simulink model "wind_turbine_modified"  (R2023a)
settings: Solver=VariableStepAuto  StartTime=0.0  StopTime=10.0  RelTol=1e-3
undefined symbols (not defined in the file): F, find_system, Fnom, gcbh, H, ILd_init, ILq_init, Imax_grid_conv, Init, j, Ki_dc_reg, Ki_grid_side_cur_reg, Ki_power_reg, Ki_Q, Ki_rotor_side_cur_reg, Ki_volt_reg, Kp_dc_reg, Kp_grid_side_cur_reg, Kp_power_reg, Kp_Q, Kp_rotor_side_cur_reg, Kp_volt_reg, L_RL, Llr, Lls, p, Pnom, power_A, power_B, power_D, R_RL, Rr, Rs, speed_A, speed_B, speed_C, speed_D, sps_rtmsupport, Vcontrol, Vnom, Wind_On
libraries: simulink_extras x5, spsControlledCurrentSourceLib x4, spsThreePhaseVIMeasurementLib x2, spsWindTurbineDoublyFedInductionGeneratorPhasorTypeLib x1, spsBistableLib x1, spsPower3phPhasorLib x1, spsWindTurbineLib x1
(part 2 of 3)

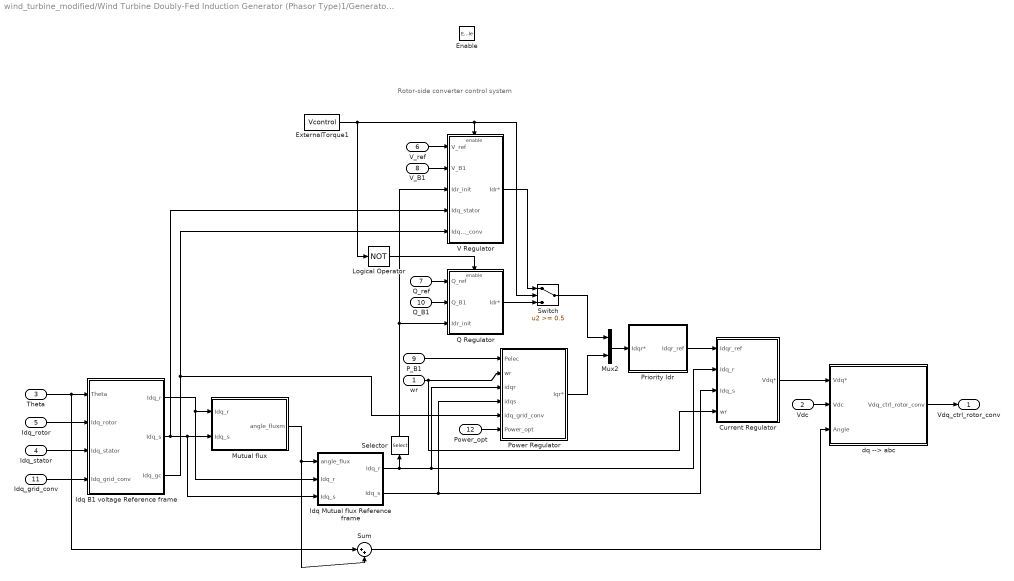
== system wind_turbine_modified/Wind Turbine Doubly-Fed Induction Generator (Phasor Type)1/Generator & Converters/Control/wind_dfig_rotor ==
  note: Rotor-side converter control system
  wr : Inport
  Vdc : Inport  Port=2
  Theta : Inport  Port=3
  Idq_stator : Inport  Port=4
  Idq_rotor : Inport  Port=5
  V_ref : Inport  Port=6
  Q_ref : Inport  Port=7
  V_B1 : Inport  Port=8
  P_B1 : Inport  Port=9
  Q_B1 : Inport  Port=10
  Idq_grid_conv : Inport  Port=11
  Power_opt : Inport  Port=12
  Enable : EnablePort  PropagateVarSize=During execution
  Current Regulator : Subsystem
  ExternalTorque1 : Constant  Value=Vcontrol
  Idq B1 voltage Reference frame : Subsystem
  Idq Mutual flux Reference frame : Subsystem
  Logical Operator : Logic  Operator=NOT  AllPortsSameDT=off
  Mutual flux : Subsystem
  Mux2 : Mux  Inputs=2
  Power Regulator : Subsystem
  Priority Idr : Subsystem
  Q Regulator : Subsystem
  Selector : Selector  InputPortWidth=2  IndexOptions=Index vector (dialog)  Indices=1  OutputSizes=1
  Sum : Sum  Inputs=|++  SaturateOnIntegerOverflow=on
  Switch : Switch  Threshold=0.5  InputSameDT=off
  V Regulator : Subsystem
  dq --> abc : Subsystem
  Vdq_ctrl_rotor_conv : Outport  VectorParamsAs1DForOutWhenUnconnected=off
  wires:
  Mutual flux/1(angle_fluxm) -> Sum/2, Idq Mutual flux Reference frame/1(angle_flux)
  wr/1 -> Current Regulator/4(wr), Power Regulator/2(wr)
  Mux2/1 -> Priority Idr/1(Idqr*)
  Current Regulator/1(Vdq*) -> dq --> abc/1(Vdq*)
  Vdc/1 -> dq --> abc/2(Vdc)
  Theta/1 -> Sum/1, Idq B1 voltage Reference frame/1(Theta)
  Idq Mutual flux Reference frame/1("Idq_r ") -> Selector/1, Current Regulator/2(Idq_r), Power Regulator/3(idqr)
  Sum/1 -> dq --> abc/3(Angle)
  dq --> abc/1(Vdq_ctrl_rotor_conv) -> Vdq_ctrl_rotor_conv/1
  Idq B1 voltage Reference frame/2(Idq_s) -> Idq Mutual flux Reference frame/3(Idq_s), Mutual flux/2(Idq_s), V Regulator/4(Idq_stator)
  Idq Mutual flux Reference frame/2("Idq_s ") -> Current Regulator/3(Idq_s), Power Regulator/4(idqs)
  Idq_rotor/1 -> Idq B1 voltage Reference frame/2(Idq_rotor)
  Idq_stator/1 -> Idq B1 voltage Reference frame/3(Idq_stator)
  Idq B1 voltage Reference frame/1(Idq_r) -> Mutual flux/1(Idq_r), Idq Mutual flux Reference frame/2(Idq_r)
  Q_ref/1 -> Q Regulator/1(Q_ref)
  Q_B1/1 -> Q Regulator/2(Q_B1)
  Selector/1 -> V Regulator/3(Idr_init), Q Regulator/3(Idr_init)
  P_B1/1 -> Power Regulator/1(Pelec)
  V_ref/1 -> V Regulator/1(V_ref)
  V_B1/1 -> V Regulator/2(V_B1)
  ExternalTorque1/1 -> Logical Operator/1, Switch/2, V Regulator/Enable
  Logical Operator/1 -> Q Regulator/Enable
  Q Regulator/1(Idr*) -> Switch/3
  V Regulator/1(Idr*) -> Switch/1
  Idq B1 voltage Reference frame/3(Idq_gc) -> V Regulator/5(Idq_grid_conv), Power Regulator/5(idq_grid_conv)
  Idq_grid_conv/1 -> Idq B1 voltage Reference frame/4(Idq_grid_conv)
  Priority Idr/1(Idqr_ref) -> Current Regulator/1(Idqr_ref)
  Power_opt/1 -> Power Regulator/6(Power_opt)
  Switch/1 -> Mux2/1
  Power Regulator/1(Iqr*) -> Mux2/2

== system wind_turbine_modified/Wind Turbine Doubly-Fed Induction Generator (Phasor Type)1/Generator & Converters/Grid-side converter currents & Converters power/d-q axis model of a 3-phase series R-L branch ==
  note: where w = 2*pi*Fnom (Hz)
  note: Vq1 - Vq2 = [ R * Iq ] + [ L* w * Id ] + [ L * d/dt (Iq) ]
  note: ==========================================================================================
  note: I --->
  note: V2
  note: V1
  note: o--------| R |---| L |-------o
  note: Vd1 - Vd2 = [ R * Id ] - [ L* w * Iq ] + [ L * d/dt (Id) ]
  note: where w = 2*pi*Fnom (Hz)
  note: Iq = [ w / ( L * s ) ] * [ Vq1 - Vq2 - ( R * Iq ) - ( L * Id ) ]
  note: Id = [ w / ( L * s ) ] * [ Vd1 - Vd2 - ( R * Id ) + ( L * Iq ) ]
  note: d-q axis model of a 3-phase series R-L branch
  note: Using Laplace transform and per unit (pu) quantities :
  Vdq1 : Inport
  Vdq2 : Inport  Port=2
  Trip : Inport  Port=3
  Constant : Constant  Value=0
  Integrator : Integrator  InitialCondition=Idq0
  R_choke : Gain  Gain=R  SaturateOnIntegerOverflow=on  OutDataTypeStr=Inherit: Same as input  ParamDataTypeStr=Inherit: Same as input
  R_choke1 : Gain  Gain=L  SaturateOnIntegerOverflow=on  OutDataTypeStr=Inherit: Same as input  ParamDataTypeStr=Inherit: Same as input
  R_choke2 : Gain  Gain=[1 -1]  SaturateOnIntegerOverflow=on  OutDataTypeStr=Inherit: Same as input  ParamDataTypeStr=Inherit: Same as input
  R_choke3 : Gain  Gain=w / L  SaturateOnIntegerOverflow=on  OutDataTypeStr=Inherit: Same as input  ParamDataTypeStr=Inherit: Same as input
  Selector : Selector  InputPortWidth=2  IndexOptions=Index vector (dialog)  Indices=[2 1]  OutputSizes=1
  Sum : Sum  Inputs=+--+  SaturateOnIntegerOverflow=on
  Switch : Switch  Criteria=u2 ~= 0  Threshold=0.5  InputSameDT=off
  Switch1 : Switch  Criteria=u2 ~= 0  Threshold=0.5  InputSameDT=off
  Idq : Outport  VectorParamsAs1DForOutWhenUnconnected=off
  wires:
  Selector/1 -> R_choke1/1
  Sum/1 -> R_choke3/1
  R_choke1/1 -> R_choke2/1
  R_choke2/1 -> Sum/4
  R_choke/1 -> Sum/3
  Vdq2/1 -> Sum/2
  Vdq1/1 -> Sum/1
  Switch/1 -> Integrator/1
  R_choke3/1 -> Switch/3
  Constant/1 -> Switch/1, Switch1/1
  Switch1/1 -> Idq/1, Selector/1, R_choke/1
  Integrator/1 -> Switch1/3
  Trip/1 -> Switch/2, Switch1/2

== system wind_turbine_modified/Wind Turbine Doubly-Fed Induction Generator (Phasor Type)1/Generator & Converters/Grid-side converter currents & Converters power/dq2ab ==
  note: Ia = I1
      | Ib = (a^2 * I1)
  Idq_seq1 : Inport
  Demux1 : Demux  Outputs=2
      settings: DisplayOption=none
  Mux : Mux  Inputs=2
  Real-Imag to Complex1 : RealImagToComplex
  a^2 : Gain  Gain=exp(-j*2*pi/3)  SaturateOnIntegerOverflow=on  OutDataTypeStr=Inherit: Same as input  ParamDataTypeStr=Inherit: Same as input
  Ia_Ib complx : Outport  VectorParamsAs1DForOutWhenUnconnected=off
  wires:
  Mux/1 -> Ia_Ib complx/1
  Idq_seq1/1 -> Demux1/1
  Demux1/1 -> Real-Imag to Complex1/1
  Demux1/2 -> Real-Imag to Complex1/2
  Real-Imag to Complex1/1 -> Mux/1, a^2/1  "I1"
  a^2/1 -> Mux/2

== system wind_turbine_modified/Wind Turbine Doubly-Fed Induction Generator (Phasor Type)1/Generator & Converters/Asynchronous machine Positive sequence phasor model Inputs and outputs are in per unit (pu)/Positive Sequence Model/Mutual fluxes ==
  phiqr,phidr : Inport
  phiqs,phids : Inport  Port=2
  1\Llr : Gain  Gain=1/Llr  SaturateOnIntegerOverflow=on  OutDataTypeStr=Inherit: Same as input  ParamDataTypeStr=Inherit: Same as input
  1\Llr1 : Gain  Gain=Laq  SaturateOnIntegerOverflow=on  OutDataTypeStr=Inherit: Same as input  ParamDataTypeStr=Inherit: Same as input
  1\Llr2 : Gain  Gain=Lad  SaturateOnIntegerOverflow=on  OutDataTypeStr=Inherit: Same as input  ParamDataTypeStr=Inherit: Same as input
  1\Lls : Gain  Gain=1/Lls  SaturateOnIntegerOverflow=on  OutDataTypeStr=Inherit: Same as input  ParamDataTypeStr=Inherit: Same as input
  Demux1 : Demux  Outputs=2
      settings: DisplayOption=none
  Demux2 : Demux  Outputs=2
      settings: DisplayOption=none
  Mux3 : Mux  Inputs=2
  Sum : Sum  Inputs=|++  InputSameDT=on  SaturateOnIntegerOverflow=on  OutDataTypeStr=Inherit: Same as first input
  Sum1 : Sum  Inputs=++|  InputSameDT=on  SaturateOnIntegerOverflow=on  OutDataTypeStr=Inherit: Same as first input
  phimq,phimd : Outport  VectorParamsAs1DForOutWhenUnconnected=off
  wires:
  Mux3/1 -> phimq,phimd/1
  1\Llr2/1 -> Mux3/2
  1\Llr1/1 -> Mux3/1
  Demux1/2 -> Sum1/1
  Demux2/2 -> Sum1/2
  Demux2/1 -> Sum/2
  1\Lls/1 -> Demux2/1
  Sum/1 -> 1\Llr1/1
  1\Llr/1 -> Demux1/1
  phiqr,phidr/1 -> 1\Llr/1
  phiqs,phids/1 -> 1\Lls/1
  Sum1/1 -> 1\Llr2/1
  Demux1/1 -> Sum/1

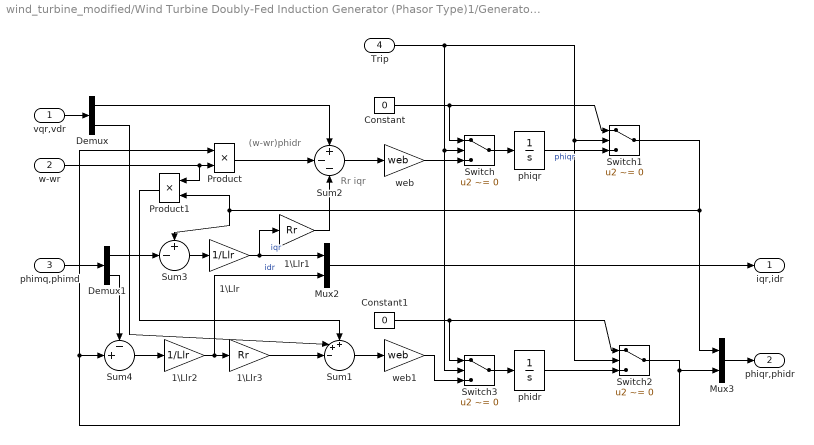
== system wind_turbine_modified/Wind Turbine Doubly-Fed Induction Generator (Phasor Type)1/Generator & Converters/Asynchronous machine Positive sequence phasor model Inputs and outputs are in per unit (pu)/Positive Sequence Model/Rotor ==
  note: Rr iqr
  note: (w-wr)phidr
  vqr,vdr : Inport
  w-wr : Inport  Port=2
  phimq,phimd : Inport  Port=3
  Trip : Inport  Port=4
  1\Llr : Gain  Gain=1/Llr  SaturateOnIntegerOverflow=on  OutDataTypeStr=Inherit: Same as input  ParamDataTypeStr=Inherit: Same as input
  1\Llr1 : Gain  Gain=Rr  SaturateOnIntegerOverflow=on  OutDataTypeStr=Inherit: Same as input  ParamDataTypeStr=Inherit: Same as input
  1\Llr2 : Gain  Gain=1/Llr  SaturateOnIntegerOverflow=on  OutDataTypeStr=Inherit: Same as input  ParamDataTypeStr=Inherit: Same as input
  1\Llr3 : Gain  Gain=Rr  SaturateOnIntegerOverflow=on  OutDataTypeStr=Inherit: Same as input  ParamDataTypeStr=Inherit: Same as input
  Constant : Constant  Value=0
  Constant1 : Constant  Value=0
  Demux : Demux  Outputs=2
      settings: DisplayOption=none
  Demux1 : Demux  Outputs=2
      settings: DisplayOption=none
  Mux2 : Mux  Inputs=2
  Mux3 : Mux  Inputs=2
  Product : Product  InputSameDT=on  SaturateOnIntegerOverflow=on  OutDataTypeStr=Inherit: Same as first input
  Product1 : Product  InputSameDT=on  SaturateOnIntegerOverflow=on  OutDataTypeStr=Inherit: Same as first input
  Sum1 : Sum  Inputs=++-||  InputSameDT=on  SaturateOnIntegerOverflow=on  OutDataTypeStr=Inherit: Same as first input
  Sum2 : Sum  Inputs=+--  InputSameDT=on  SaturateOnIntegerOverflow=on  OutDataTypeStr=Inherit: Same as first input
  Sum3 : Sum  Inputs=+-|  InputSameDT=on  SaturateOnIntegerOverflow=on  OutDataTypeStr=Inherit: Same as first input
  Sum4 : Sum  Inputs=-+|  InputSameDT=on  SaturateOnIntegerOverflow=on  OutDataTypeStr=Inherit: Same as first input
  Switch{,1..3} (4 alike) : Switch  Criteria=u2 ~= 0  Threshold=0.5  InputSameDT=off
  phidr : Integrator  InitialCondition=phirdo
  phiqr : Integrator  InitialCondition=phirqo
  web : Gain  Gain=web  SaturateOnIntegerOverflow=on  OutDataTypeStr=Inherit: Same as input  ParamDataTypeStr=Inherit: Same as input
  web1 : Gain  Gain=web  SaturateOnIntegerOverflow=on  OutDataTypeStr=Inherit: Same as input  ParamDataTypeStr=Inherit: Same as input
  iqr,idr : Outport  VectorParamsAs1DForOutWhenUnconnected=off
  phiqr,phidr : Outport  Port=2  VectorParamsAs1DForOutWhenUnconnected=off
  wires:
  Mux3/1 -> phiqr,phidr/1
  Sum1/1 -> web1/1
  w-wr/1 -> Product/2, Product1/1
  Product/1 -> Sum2/2
  Sum2/1 -> web/1
  phidr/1 -> Switch2/3
  vqr,vdr/1 -> Demux/1
  Product1/1 -> Sum1/1
  Demux/2 -> Sum1/2
  1\Llr3/1 -> Sum1/3
  1\Llr2/1 -> 1\Llr3/1, Mux2/2  "idr"
  Sum4/1 -> 1\Llr2/1
  Demux1/2 -> Sum4/1
  Mux2/1 -> iqr,idr/1
  1\Llr/1 -> Mux2/1, 1\Llr1/1  "iqr"
  1\Llr1/1 -> Sum2/3
  Sum3/1 -> 1\Llr/1
  Demux/1 -> Sum2/1
  Demux1/1 -> Sum3/2
  phimq,phimd/1 -> Demux1/1
  web/1 -> Switch/3
  Switch/1 -> phiqr/1
  Constant/1 -> Switch/1, Switch1/1
  Switch1/1 -> Mux3/1, Product1/2, Sum3/1
  phiqr/1 -> Switch1/3  "phiqr"
  Switch2/1 -> Mux3/2, Sum4/2, Product/1
  Switch3/1 -> phidr/1
  web1/1 -> Switch3/3
  Constant1/1 -> Switch2/1, Switch3/1
  Trip/1 -> Switch/2, Switch3/2, Switch1/2, Switch2/2

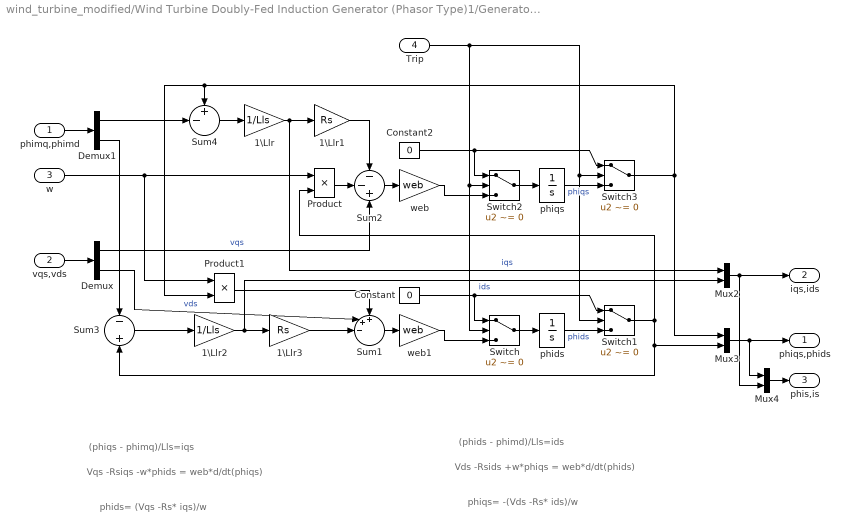
== system wind_turbine_modified/Wind Turbine Doubly-Fed Induction Generator (Phasor Type)1/Generator & Converters/Asynchronous machine Positive sequence phasor model Inputs and outputs are in per unit (pu)/Positive Sequence Model/Stator ==
  note: phids= (Vqs -Rs* iqs)/w
  note: phiqs= -(Vds -Rs* ids)/w
  note: Vqs -Rsiqs -w*phids = web*d/dt(phiqs)
  note: (phiqs - phimq)/Lls=iqs
  note: Vds -Rsids +w*phiqs = web*d/dt(phids)
  note: (phids - phimd)/Lls=ids
  phimq,phimd : Inport
  vqs,vds : Inport  Port=2
  w : Inport  Port=3
  Trip : Inport  Port=4
  1\Llr : Gain  Gain=1/Lls  SaturateOnIntegerOverflow=on  OutDataTypeStr=Inherit: Same as input  ParamDataTypeStr=Inherit: Same as input
  1\Llr1 : Gain  Gain=Rs  SaturateOnIntegerOverflow=on  OutDataTypeStr=Inherit: Same as input  ParamDataTypeStr=Inherit: Same as input
  1\Llr2 : Gain  Gain=1/Lls  SaturateOnIntegerOverflow=on  OutDataTypeStr=Inherit: Same as input  ParamDataTypeStr=Inherit: Same as input
  1\Llr3 : Gain  Gain=Rs  SaturateOnIntegerOverflow=on  OutDataTypeStr=Inherit: Same as input  ParamDataTypeStr=Inherit: Same as input
  Constant : Constant  Value=0
  Constant2 : Constant  Value=0
  Demux : Demux  Outputs=2
      settings: DisplayOption=none
  Demux1 : Demux  Outputs=2
      settings: DisplayOption=none
  Mux2 : Mux  Inputs=2
  Mux3 : Mux  Inputs=2
  Mux4 : Mux  Inputs=2
  Product : Product  InputSameDT=on  SaturateOnIntegerOverflow=on  OutDataTypeStr=Inherit: Same as first input
  Product1 : Product  InputSameDT=on  SaturateOnIntegerOverflow=on  OutDataTypeStr=Inherit: Same as first input
  Sum1 : Sum  Inputs=++-||  InputSameDT=on  SaturateOnIntegerOverflow=on  OutDataTypeStr=Inherit: Same as first input
  Sum2 : Sum  Inputs=--+  InputSameDT=on  SaturateOnIntegerOverflow=on  OutDataTypeStr=Inherit: Same as first input
  Sum3 : Sum  Inputs=-+  InputSameDT=on  SaturateOnIntegerOverflow=on  OutDataTypeStr=Inherit: Same as first input
  Sum4 : Sum  Inputs=+-|  InputSameDT=on  SaturateOnIntegerOverflow=on  OutDataTypeStr=Inherit: Same as first input
  Switch{,1..3} (4 alike) : Switch  Criteria=u2 ~= 0  Threshold=0.5  InputSameDT=off
  phids : Integrator  InitialCondition=phisdo
  phiqs : Integrator  InitialCondition=phisqo
  web : Gain  Gain=web  SaturateOnIntegerOverflow=on  OutDataTypeStr=Inherit: Same as input  ParamDataTypeStr=Inherit: Same as input
  web1 : Gain  Gain=web  SaturateOnIntegerOverflow=on  OutDataTypeStr=Inherit: Same as input  ParamDataTypeStr=Inherit: Same as input
  phiqs,phids : Outport  VectorParamsAs1DForOutWhenUnconnected=off
  iqs,ids : Outport  Port=2  VectorParamsAs1DForOutWhenUnconnected=off
  phis,is : Outport  Port=3  VectorParamsAs1DForOutWhenUnconnected=off
  wires:
  Demux/1 -> Sum2/3  "vqs"
  Mux2/1 -> iqs,ids/1, Mux4/2
  1\Llr2/1 -> 1\Llr3/1, Mux2/2  "ids"
  1\Llr3/1 -> Sum1/3
  Sum1/1 -> web1/1
  Demux/2 -> Sum1/2  "vds"
  Product1/1 -> Sum1/1
  Mux3/1 -> phiqs,phids/1, Mux4/1
  Mux4/1 -> phis,is/1
  Sum4/1 -> 1\Llr/1
  1\Llr/1 -> Mux2/1, 1\Llr1/1  "iqs"
  1\Llr1/1 -> Sum2/1
  Sum2/1 -> web/1
  Product/1 -> Sum2/2
  phiqs/1 -> Switch3/3  "phiqs"
  vqs,vds/1 -> Demux/1
  Demux1/2 -> Sum3/1
  Sum3/1 -> 1\Llr2/1
  phimq,phimd/1 -> Demux1/1
  Demux1/1 -> Sum4/2
  w/1 -> Product/1, Product1/1
  Switch/1 -> phids/1
  web1/1 -> Switch/3
  Constant/1 -> Switch/1, Switch1/1
  phids/1 -> Switch1/3  "phids"
  Switch1/1 -> Product/2, Mux3/2, Sum3/2
  Switch2/1 -> phiqs/1
  web/1 -> Switch2/3
  Constant2/1 -> Switch2/1, Switch3/1
  Switch3/1 -> Sum4/1, Product1/2, Mux3/1
  Trip/1 -> Switch2/2, Switch/2, Switch3/2, Switch1/2

== system wind_turbine_modified/Wind Turbine Doubly-Fed Induction Generator (Phasor Type)1/Generator & Converters/Control/wind_dfig_grid/Current regulator ==
  Vdq : Inport
  Idq : Inport  Port=2
  Idq_ref : Inport  Port=3
  Constant1 : Constant  Value=L_RL
  Constant2 : Constant  Value=L_RL
  Constant3 : Constant  Value=R_RL
  Constant4 : Constant  Value=R_RL
  Demux{,1..3} (4 alike) : Demux  Outputs=2
      settings: DisplayOption=none
  Mux : Mux  Inputs=2
  Mux1 : Mux  Inputs=2
  Product{,1..3} (4 alike) : Product  InputSameDT=on  SaturateOnIntegerOverflow=on  OutDataTypeStr=Inherit: Same as first input
  Subsystem3 : Subsystem  mask{Kp=Kp_grid_side_cur_reg, Ki=Ki_grid_side_cur_reg, Limits=[inf -inf], Init=0}
      mask prompts: Kp "Proportional gain (Kp):"; Ki "Integral gain (Ki):"; Limits "Output limits [Upper Lower]:"; Init "Output initial value:"
      mask init:
      | Upper_Limit=Limits(1);
      | Lower_Limit=Limits(2);
      mask Display: disp('PI')
  Sum1 : Sum  Inputs=|+-  InputSameDT=on  SaturateOnIntegerOverflow=on  OutDataTypeStr=Inherit: Same as first input
  Sum2 : Sum  Inputs=-+|  InputSameDT=on  SaturateOnIntegerOverflow=on  OutDataTypeStr=Inherit: Same as first input
  Sum3 : Sum  Inputs=||++-  InputSameDT=on  SaturateOnIntegerOverflow=on  OutDataTypeStr=Inherit: Same as first input
  Sum4 : Sum  Inputs=|+-  InputSameDT=on  SaturateOnIntegerOverflow=on  OutDataTypeStr=Inherit: Same as first input
  Sum5 : Sum  Inputs=|--+  InputSameDT=on  SaturateOnIntegerOverflow=on  OutDataTypeStr=Inherit: Same as first input
  Sum6 : Sum  Inputs=|-+  InputSameDT=on  SaturateOnIntegerOverflow=on  OutDataTypeStr=Inherit: Same as first input
  Vdq* : Outport  VectorParamsAs1DForOutWhenUnconnected=off
  wires:
  Product3/1 -> Sum5/1
  Product2/1 -> Sum3/3
  Demux2/2 -> Sum5/3  "Vq"
  Product1/1 -> Sum5/2
  Constant4/1 -> Product3/2
  Constant3/1 -> Product2/1
  Sum4/1 -> Mux1/1
  Product/1 -> Sum3/2
  Demux3/2 -> Sum6/1  "vq'"
  Mux/1 -> Vdq*/1
  Sum1/1 -> Mux/1
  Sum6/1 -> Mux/2
  Idq/1 -> Demux/1
  Demux/1 -> Product2/2, Sum4/2, Product1/1  "Id"
  Demux/2 -> Product3/1, Sum2/1, Product/2  "Iq"
  Sum2/1 -> Mux1/2
  Demux1/1 -> Sum4/1  "Id_ref"
  Idq_ref/1 -> Demux1/1
  Demux1/2 -> Sum2/2  "Iq_ref"
  Vdq/1 -> Demux2/1
  Constant1/1 -> Product/1
  Demux2/1 -> Sum3/1  "Vd"
  Sum3/1 -> Sum1/1
  Sum5/1 -> Sum6/2
  Mux1/1 -> Subsystem3/1(In1)
  Subsystem3/1(Out1) -> Demux3/1
  Demux3/1 -> Sum1/2  "vd'"
  Constant2/1 -> Product1/2

== system wind_turbine_modified/Wind Turbine Doubly-Fed Induction Generator (Phasor Type)1/Generator & Converters/Control/wind_dfig_grid/DC bus voltage Regulator ==
  Vdc_ref : Inport
  Vdc : Inport  Port=2
  Rate Limiter : RateLimiter  RisingSlewLimit=current_slew_rate  FallingSlewLimit=-current_slew_rate
  Subsystem1 : Subsystem  mask{Kp=Kp_dc_reg, Ki=Ki_dc_reg, Limits=[1 -1]*Imax_grid_conv, Init=ILd_init}
      mask prompts: Kp "Proportional gain (Kp):"; Ki "Integral gain (Ki):"; Limits "Output limits [Upper Lower]:"; Init "Output initial value:"
      mask init:
      | Upper_Limit=Limits(1);
      | Lower_Limit=Limits(2);
      mask Display: disp('PI')
  Sum7 : Sum  Inputs=|+-  InputSameDT=on  SaturateOnIntegerOverflow=on  OutDataTypeStr=Inherit: Same as first input
  Id_ref : Outport  VectorParamsAs1DForOutWhenUnconnected=off
  wires:
  Sum7/1 -> Subsystem1/1(In1)
  Vdc_ref/1 -> Sum7/1
  Subsystem1/1(Out1) -> Rate Limiter/1
  Vdc/1 -> Sum7/2
  Rate Limiter/1 -> Id_ref/1

== system wind_turbine_modified/Wind Turbine Doubly-Fed Induction Generator (Phasor Type)1/Generator & Converters/Control/wind_dfig_grid/Idq B1 voltage Reference frame ==
  Theta : Inport
  Idq_grid_conv : Inport  Port=2
  Complex to Magnitude-Angle : ComplexToMagnitudeAngle
  Complex to Real-Imag : ComplexToRealImag
  Demux1 : Demux  Outputs=2
      settings: DisplayOption=none
  Magnitude-Angle to Complex : MagnitudeAngleToComplex
  Mux : Mux  Inputs=2
  Real-Imag to Complex : RealImagToComplex
  Sum : Sum  Inputs=|+-  SaturateOnIntegerOverflow=on
  Idq : Outport  VectorParamsAs1DForOutWhenUnconnected=off
  wires:
  Theta/1 -> Sum/2
  Real-Imag to Complex/1 -> Complex to Magnitude-Angle/1
  Demux1/2 -> Real-Imag to Complex/2
  Demux1/1 -> Real-Imag to Complex/1
  Idq_grid_conv/1 -> Demux1/1
  Mux/1 -> Idq/1
  Complex to Magnitude-Angle/2 -> Sum/1
  Complex to Magnitude-Angle/1 -> Magnitude-Angle to Complex/1
  Sum/1 -> Magnitude-Angle to Complex/2
  Magnitude-Angle to Complex/1 -> Complex to Real-Imag/1
  Complex to Real-Imag/1 -> Mux/1  "Id"
  Complex to Real-Imag/2 -> Mux/2  "Iq"

== system wind_turbine_modified/Wind Turbine Doubly-Fed Induction Generator (Phasor Type)1/Generator & Converters/Control/wind_dfig_grid/Idq references ==
  Id*Iq* : Inport
  Cartesian to Polar : simulink_extras/Transformations/Cartesian to Polar
  Demux : Demux  Outputs=2
      settings: DisplayOption=none
  Igrid_conv_max^2 : Constant  Value=Imax_grid_conv*Imax_grid_conv
  Math Function : Math  Operator=square  SignedPower=on
  Math Function1 : Math  Operator=sqrt  SignedPower=on
  Mux : Mux  Inputs=2
  Mux1 : Mux  Inputs=2
  Product : Product  InputSameDT=on  SaturateOnIntegerOverflow=on  OutDataTypeStr=Inherit: Same as first input
  Rate Limiter : RateLimiter  RisingSlewLimit=current_slew_rate  FallingSlewLimit=-current_slew_rate
  Sign : Signum  ZeroCross=off
  Sum : Sum  Inputs=|+-  InputSameDT=on  SaturateOnIntegerOverflow=on  OutDataTypeStr=Inherit: Same as first input
  Switch : Switch  Threshold=Imax_grid_conv
  Terminator : Terminator
  Idq_ref : Outport  VectorParamsAs1DForOutWhenUnconnected=off
  wires:
  Product/1 -> Mux1/2
  Rate Limiter/1 -> Idq_ref/1
  Demux/2 -> Cartesian to Polar/2, Mux/2, Sign/1
  Demux/1 -> Mux1/1, Math Function/1, Cartesian to Polar/1, Mux/1
  Cartesian to Polar/2 -> Terminator/1
  Cartesian to Polar/1 -> Switch/2
  Mux/1 -> Switch/3
  Igrid_conv_max^2/1 -> Sum/1
  Math Function/1 -> Sum/2
  Sum/1 -> Math Function1/1
  Mux1/1 -> Switch/1
  Switch/1 -> Rate Limiter/1
  Math Function1/1 -> Product/2  "Iq"
  Sign/1 -> Product/1
  Id*Iq*/1 -> Demux/1

== system wind_turbine_modified/Wind Turbine Doubly-Fed Induction Generator (Phasor Type)1/Generator & Converters/Control/wind_dfig_grid/Subsystem ==
  note: Required value for modulation index "m" to obtain 1 pu generated voltage by the converter:
  note: m = Vnom * 2*sqrt(2/3) / Vdc
  note: Where Vnom = RMS ph-ph nominal voltage
  Theta : Inport
  Vdq* : Inport  Port=2
  Vdc : Inport  Port=3
  0-1 : Saturate  UpperLimit=1  LowerLimit=0
  Avoid division by zero : Saturate  UpperLimit=1e6  LowerLimit=1e-6
  Cartesian to Polar1 : simulink_extras/Transformations/Cartesian to Polar
  Demux1 : Demux  Outputs=2
      settings: DisplayOption=none
  K : Constant  Value=Vnom*2*sqrt(2/3)
  Magnitude-Angle to Complex : MagnitudeAngleToComplex
  Product1 : Product  Inputs=**/  InputSameDT=on  SaturateOnIntegerOverflow=on  OutDataTypeStr=Inherit: Same as first input
  Sum : Sum  Inputs=|++  SaturateOnIntegerOverflow=on
  Vdq_ctrl_grid_conv : Outport  VectorParamsAs1DForOutWhenUnconnected=off
  wires:
  Theta/1 -> Sum/2
  Magnitude-Angle to Complex/1 -> Vdq_ctrl_grid_conv/1
  Sum/1 -> Magnitude-Angle to Complex/2
  0-1/1 -> Magnitude-Angle to Complex/1
  Product1/1 -> 0-1/1  "m"
  Vdc/1 -> Avoid division by zero/1
  K/1 -> Product1/2
  Avoid division by zero/1 -> Product1/3
  Vdq*/1 -> Demux1/1
  Demux1/1 -> Cartesian to Polar1/1
  Demux1/2 -> Cartesian to Polar1/2
  Cartesian to Polar1/1 -> Product1/1
  Cartesian to Polar1/2 -> Sum/1

== system wind_turbine_modified/Wind Turbine Doubly-Fed Induction Generator (Phasor Type)1/Generator & Converters/Control/wind_dfig_grid/Vdq B1 voltage Reference frame ==
  Theta : Inport
  Vdq_B1 : Inport  Port=2
  Complex to Magnitude-Angle : ComplexToMagnitudeAngle
  Complex to Real-Imag : ComplexToRealImag
  Demux1 : Demux  Outputs=2
      settings: DisplayOption=none
  Magnitude-Angle to Complex : MagnitudeAngleToComplex
  Mux : Mux  Inputs=2
  Real-Imag to Complex : RealImagToComplex
  Sum : Sum  Inputs=|+-  SaturateOnIntegerOverflow=on
  Vdq : Outport  VectorParamsAs1DForOutWhenUnconnected=off
  wires:
  Theta/1 -> Sum/2
  Real-Imag to Complex/1 -> Complex to Magnitude-Angle/1
  Demux1/2 -> Real-Imag to Complex/2
  Demux1/1 -> Real-Imag to Complex/1
  Vdq_B1/1 -> Demux1/1
  Mux/1 -> Vdq/1
  Complex to Magnitude-Angle/2 -> Sum/1
  Complex to Magnitude-Angle/1 -> Magnitude-Angle to Complex/1
  Sum/1 -> Magnitude-Angle to Complex/2
  Magnitude-Angle to Complex/1 -> Complex to Real-Imag/1
  Complex to Real-Imag/1 -> Mux/1  "Vd"
  Complex to Real-Imag/2 -> Mux/2  "Vq"

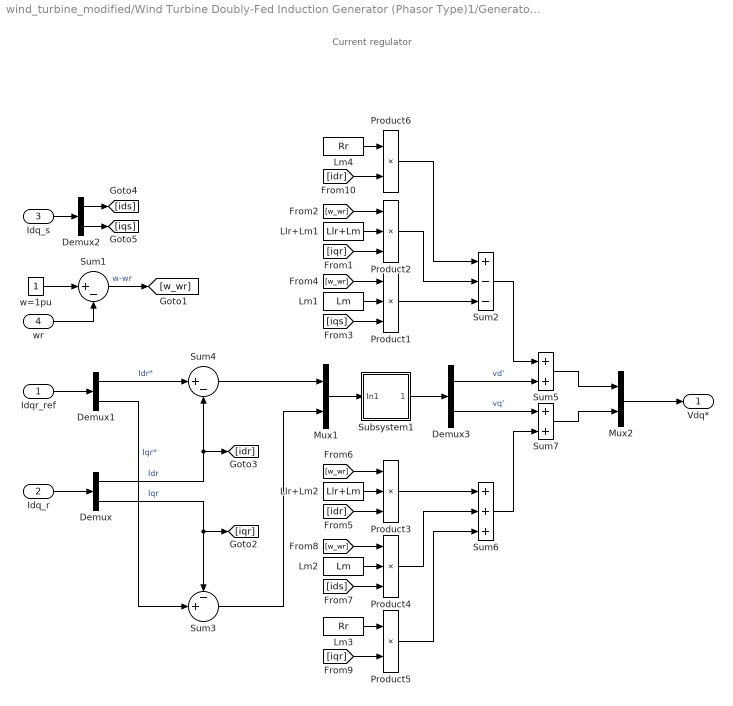
== system wind_turbine_modified/Wind Turbine Doubly-Fed Induction Generator (Phasor Type)1/Generator & Converters/Control/wind_dfig_rotor/Current Regulator ==
  note: Current regulator
  Idqr_ref : Inport
  Idq_r : Inport  Port=2
  Idq_s : Inport  Port=3
  wr : Inport  Port=4
  Demux{,1..3} (4 alike) : Demux  Outputs=2
      settings: DisplayOption=none
  Llr+Lm1 : Constant  Value=Llr+Lm
  Llr+Lm2 : Constant  Value=Llr+Lm
  Lm1 : Constant  Value=Lm
  Lm2 : Constant  Value=Lm
  Lm3 : Constant  Value=Rr
  Lm4 : Constant  Value=Rr
  Mux1 : Mux  Inputs=2
  Mux2 : Mux  Inputs=2
  Product{1..4} (4 alike) : Product  Inputs=3  SaturateOnIntegerOverflow=on  OutDataTypeStr=Inherit: Same as first input
  Product5 : Product  SaturateOnIntegerOverflow=on  OutDataTypeStr=Inherit: Same as first input
  Product6 : Product  SaturateOnIntegerOverflow=on  OutDataTypeStr=Inherit: Same as first input
  Subsystem1 : Subsystem  mask{Kp=Kp_rotor_side_cur_reg, Ki=Ki_rotor_side_cur_reg, Limits=[inf -inf], Init=0}
      mask prompts: Kp "Proportional gain (Kp):"; Ki "Integral gain (Ki):"; Limits "Output limits [Upper Lower]:"; Init "Output initial value:"
      mask init:
      | Upper_Limit=Limits(1);
      | Lower_Limit=Limits(2);
      mask Display: disp('PI')
  Sum1 : Sum  Inputs=|+-  InputSameDT=on  SaturateOnIntegerOverflow=on  OutDataTypeStr=Inherit: Same as first input
  Sum2 : Sum  Inputs=+--  InputSameDT=on  SaturateOnIntegerOverflow=on  OutDataTypeStr=Inherit: Same as first input
  Sum3 : Sum  Inputs=-+|  InputSameDT=on  SaturateOnIntegerOverflow=on  OutDataTypeStr=Inherit: Same as first input
  Sum4 : Sum  Inputs=|+-  InputSameDT=on  SaturateOnIntegerOverflow=on  OutDataTypeStr=Inherit: Same as first input
  Sum5 : Sum  InputSameDT=on  SaturateOnIntegerOverflow=on  OutDataTypeStr=Inherit: Same as first input
  Sum6 : Sum  Inputs=+++  InputSameDT=on  SaturateOnIntegerOverflow=on  OutDataTypeStr=Inherit: Same as first input
  Sum7 : Sum  InputSameDT=on  SaturateOnIntegerOverflow=on  OutDataTypeStr=Inherit: Same as first input
  w=1pu : Constant
  Vdq* : Outport  VectorParamsAs1DForOutWhenUnconnected=off
  wires:
  Idq_r/1 -> Demux/1
  Demux/1 -> Sum4/2, [idr]  "Idr"
  Demux/2 -> Sum3/1, [iqr]  "Iqr"
  Sum4/1 -> Mux1/1
  Sum3/1 -> Mux1/2
  Idqr_ref/1 -> Demux1/1
  Demux1/1 -> Sum4/1  "Idr*"
  Demux1/2 -> Sum3/2  "Iqr*"
  Mux1/1 -> Subsystem1/1(In1)
  Idq_s/1 -> Demux2/1
  Subsystem1/1(Out1) -> Demux3/1
  w=1pu/1 -> Sum1/1
  wr/1 -> Sum1/2
  Demux3/1 -> Sum5/2  "vd'"
  Demux2/1 -> [ids]
  Demux2/2 -> [iqs]
  Sum1/1 -> [w_wr]  "w-wr"
  [iqr] -> Product2/3
  [w_wr] -> Product2/1
  Llr+Lm1/1 -> Product2/2
  [iqs] -> Product1/3
  [w_wr] -> Product1/1
  Lm1/1 -> Product1/2
  [idr] -> Product3/3
  [w_wr] -> Product3/1
  Llr+Lm2/1 -> Product3/2
  [ids] -> Product4/3
  [w_wr] -> Product4/1
  Lm2/1 -> Product4/2
  Product3/1 -> Sum6/1
  Demux3/2 -> Sum7/1  "vq'"
  Sum5/1 -> Mux2/1
  Sum7/1 -> Mux2/2
  Mux2/1 -> Vdq*/1
  Product4/1 -> Sum6/2
  Sum6/1 -> Sum7/2
  Sum2/1 -> Sum5/1
  Lm3/1 -> Product5/1
  [iqr] -> Product5/2
  Lm4/1 -> Product6/1
  [idr] -> Product6/2
  Product2/1 -> Sum2/2
  Product1/1 -> Sum2/3
  Product6/1 -> Sum2/1
  Product5/1 -> Sum6/3

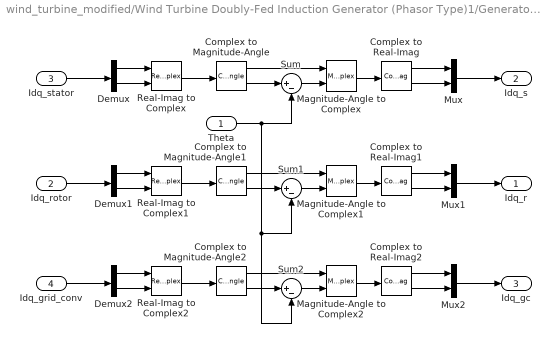
== system wind_turbine_modified/Wind Turbine Doubly-Fed Induction Generator (Phasor Type)1/Generator & Converters/Control/wind_dfig_rotor/Idq B1 voltage Reference frame ==
  Theta : Inport
  Idq_rotor : Inport  Port=2
  Idq_stator : Inport  Port=3
  Idq_grid_conv : Inport  Port=4
  Complex to Magnitude-Angle : ComplexToMagnitudeAngle
  Complex to Magnitude-Angle1 : ComplexToMagnitudeAngle
  Complex to Magnitude-Angle2 : ComplexToMagnitudeAngle
  Complex to Real-Imag : ComplexToRealImag
  Complex to Real-Imag1 : ComplexToRealImag
  Complex to Real-Imag2 : ComplexToRealImag
  Demux : Demux  Outputs=2
      settings: DisplayOption=none
  Demux1 : Demux  Outputs=2
      settings: DisplayOption=none
  Demux2 : Demux  Outputs=2
      settings: DisplayOption=none
  Magnitude-Angle to Complex : MagnitudeAngleToComplex
  Magnitude-Angle to Complex1 : MagnitudeAngleToComplex
  Magnitude-Angle to Complex2 : MagnitudeAngleToComplex
  Mux : Mux  Inputs=2
  Mux1 : Mux  Inputs=2
  Mux2 : Mux  Inputs=2
  Real-Imag to Complex : RealImagToComplex
  Real-Imag to Complex1 : RealImagToComplex
  Real-Imag to Complex2 : RealImagToComplex
  Sum : Sum  Inputs=|+-  SaturateOnIntegerOverflow=on
  Sum1 : Sum  Inputs=|+-  SaturateOnIntegerOverflow=on
  Sum2 : Sum  Inputs=|+-  SaturateOnIntegerOverflow=on
  Idq_r : Outport  VectorParamsAs1DForOutWhenUnconnected=off
  Idq_s : Outport  Port=2  VectorParamsAs1DForOutWhenUnconnected=off
  Idq_gc : Outport  Port=3  VectorParamsAs1DForOutWhenUnconnected=off
  wires:
  Complex to Real-Imag/2 -> Mux/2
  Complex to Real-Imag/1 -> Mux/1
  Magnitude-Angle to Complex/1 -> Complex to Real-Imag/1
  Sum/1 -> Magnitude-Angle to Complex/2
  Complex to Magnitude-Angle/1 -> Magnitude-Angle to Complex/1
  Complex to Magnitude-Angle/2 -> Sum/1
  Real-Imag to Complex/1 -> Complex to Magnitude-Angle/1
  Mux/1 -> Idq_s/1
  Demux/1 -> Real-Imag to Complex/1
  Demux/2 -> Real-Imag to Complex/2
  Idq_stator/1 -> Demux/1
  Complex to Real-Imag1/2 -> Mux1/2
  Complex to Real-Imag1/1 -> Mux1/1
  Magnitude-Angle to Complex1/1 -> Complex to Real-Imag1/1
  Sum1/1 -> Magnitude-Angle to Complex1/2
  Complex to Magnitude-Angle1/1 -> Magnitude-Angle to Complex1/1
  Complex to Magnitude-Angle1/2 -> Sum1/1
  Real-Imag to Complex1/1 -> Complex to Magnitude-Angle1/1
  Mux1/1 -> Idq_r/1
  Demux1/1 -> Real-Imag to Complex1/1
  Demux1/2 -> Real-Imag to Complex1/2
  Idq_rotor/1 -> Demux1/1
  Theta/1 -> Sum/2, Sum1/2, Sum2/2
  Complex to Real-Imag2/2 -> Mux2/2
  Complex to Real-Imag2/1 -> Mux2/1
  Magnitude-Angle to Complex2/1 -> Complex to Real-Imag2/1
  Sum2/1 -> Magnitude-Angle to Complex2/2
  Complex to Magnitude-Angle2/1 -> Magnitude-Angle to Complex2/1
  Complex to Magnitude-Angle2/2 -> Sum2/1
  Real-Imag to Complex2/1 -> Complex to Magnitude-Angle2/1
  Mux2/1 -> Idq_gc/1
  Demux2/1 -> Real-Imag to Complex2/1
  Demux2/2 -> Real-Imag to Complex2/2
  Idq_grid_conv/1 -> Demux2/1

== system wind_turbine_modified/Wind Turbine Doubly-Fed Induction Generator (Phasor Type)1/Generator & Converters/Control/wind_dfig_rotor/Idq Mutual flux Reference frame ==
  angle_flux : Inport
  Idq_r : Inport  Port=2
  Idq_s : Inport  Port=3
  Complex to Magnitude-Angle : ComplexToMagnitudeAngle
  Complex to Magnitude-Angle1 : ComplexToMagnitudeAngle
  Complex to Real-Imag : ComplexToRealImag
  Complex to Real-Imag1 : ComplexToRealImag
  Demux : Demux  Outputs=2
      settings: DisplayOption=none
  Demux1 : Demux  Outputs=2
      settings: DisplayOption=none
  Magnitude-Angle to Complex : MagnitudeAngleToComplex
  Magnitude-Angle to Complex1 : MagnitudeAngleToComplex
  Mux : Mux  Inputs=2
  Mux1 : Mux  Inputs=2
  Real-Imag to Complex : RealImagToComplex
  Real-Imag to Complex1 : RealImagToComplex
  Sum : Sum  Inputs=|+-  SaturateOnIntegerOverflow=on
  Sum1 : Sum  Inputs=|+-  SaturateOnIntegerOverflow=on
  "Idq_r " : Outport  VectorParamsAs1DForOutWhenUnconnected=off
  "Idq_s " : Outport  Port=2  VectorParamsAs1DForOutWhenUnconnected=off
  wires:
  Complex to Real-Imag/2 -> Mux/2
  Complex to Real-Imag/1 -> Mux/1
  Mux/1 -> "Idq_r "/1
  Complex to Magnitude-Angle/2 -> Sum/1
  angle_flux/1 -> Sum/2, Sum1/2
  Complex to Magnitude-Angle/1 -> Magnitude-Angle to Complex/1
  Sum/1 -> Magnitude-Angle to Complex/2
  Magnitude-Angle to Complex/1 -> Complex to Real-Imag/1
  Idq_r/1 -> Demux/1
  Demux/1 -> Real-Imag to Complex/1
  Demux/2 -> Real-Imag to Complex/2
  Real-Imag to Complex/1 -> Complex to Magnitude-Angle/1
  Complex to Real-Imag1/2 -> Mux1/2
  Complex to Real-Imag1/1 -> Mux1/1
  Mux1/1 -> "Idq_s "/1
  Complex to Magnitude-Angle1/2 -> Sum1/1
  Complex to Magnitude-Angle1/1 -> Magnitude-Angle to Complex1/1
  Sum1/1 -> Magnitude-Angle to Complex1/2
  Magnitude-Angle to Complex1/1 -> Complex to Real-Imag1/1
  Idq_s/1 -> Demux1/1
  Demux1/1 -> Real-Imag to Complex1/1
  Demux1/2 -> Real-Imag to Complex1/2
  Real-Imag to Complex1/1 -> Complex to Magnitude-Angle1/1

== system wind_turbine_modified/Wind Turbine Doubly-Fed Induction Generator (Phasor Type)1/Generator & Converters/Control/wind_dfig_rotor/Mutual flux ==
  Idq_r : Inport
  Idq_s : Inport  Port=2
  20% : Switch  Threshold=0.5  InputSameDT=off
  Cartesian to Polar : simulink_extras/Transformations/Cartesian to Polar
  Constant1 : Constant  Value=Lm
  Demux : Demux  Outputs=2
      settings: DisplayOption=none
  Demux1 : Demux  Outputs=2
      settings: DisplayOption=none
  IC=ic : Memory  InitialCondition=-pi/2  InheritSampleTime=on
  Product1 : Product  InputSameDT=on  SaturateOnIntegerOverflow=on  OutDataTypeStr=Inherit: Same as first input
  Product5 : Product  InputSameDT=on  SaturateOnIntegerOverflow=on  OutDataTypeStr=Inherit: Same as first input
  Relay : Relay  OnSwitchValue=0.5  OffSwitchValue=0.1
  Sum1 : Sum  InputSameDT=on  SaturateOnIntegerOverflow=on  OutDataTypeStr=Inherit: Same as first input
  Sum2 : Sum  InputSameDT=on  SaturateOnIntegerOverflow=on  OutDataTypeStr=Inherit: Same as first input
  angle_fluxm : Outport  VectorParamsAs1DForOutWhenUnconnected=off
  wires:
  Cartesian to Polar/1 -> Relay/1  "mod_phi"
  Product5/1 -> Cartesian to Polar/2  "phiqm"
  Demux1/1 -> Sum1/1
  Demux/1 -> Sum1/2
  Sum1/1 -> Product1/2  "idm"
  Demux1/2 -> Sum2/1
  Demux/2 -> Sum2/2
  Sum2/1 -> Product5/2  "iqm"
  Constant1/1 -> Product1/1, Product5/1
  Product1/1 -> Cartesian to Polar/1  "phidm"
  Idq_s/1 -> Demux1/1
  Idq_r/1 -> Demux/1
  IC=ic/1 -> 20%/3
  20%/1 -> IC=ic/1, angle_fluxm/1
  Relay/1 -> 20%/2
  Cartesian to Polar/2 -> 20%/1  "angle_phi"

== system wind_turbine_modified/Wind Turbine Doubly-Fed Induction Generator (Phasor Type)1/Generator & Converters/Control/wind_dfig_rotor/Power Regulator ==
  Pelec : Inport
  wr : Inport  Port=2
  idqr : Inport  Port=3
  idqs : Inport  Port=4
  idq_grid_conv : Inport  Port=5
  Power_opt : Inport  Port=6
  ExternalTorque : Constant  Value=Wind_On
  Logical Operator : Logic  Operator=NOT  AllPortsSameDT=off
  Rate Limiter : RateLimiter  RisingSlewLimit=current_slew_rate  FallingSlewLimit=-current_slew_rate
  Saturation : Saturate  UpperLimit=1  LowerLimit=0
  Subsystem : Subsystem
  "Subsystem " : Subsystem
  Switch : Switch  Threshold=0.5  InputSameDT=off
  Iqr* : Outport  VectorParamsAs1DForOutWhenUnconnected=off
  wires:
  Logical Operator/1 -> "Subsystem "/Enable
  wr/1 -> Subsystem/2(wr)
  Pelec/1 -> Subsystem/1(Pelec), "Subsystem "/1(Pelec)
  Saturation/1 -> Rate Limiter/1
  Switch/1 -> Saturation/1
  ExternalTorque/1 -> Switch/2, Subsystem/Enable, Logical Operator/1
  Subsystem/1(Iqr*) -> Switch/1
  "Subsystem "/1(Iqr*) -> Switch/3
  Rate Limiter/1 -> Iqr*/1
  idqs/1 -> Subsystem/3(idqs)
  idqr/1 -> Subsystem/4(idqr), "Subsystem "/2(idqr)
  idq_grid_conv/1 -> Subsystem/5(idq_grid_conv)
  Power_opt/1 -> "Subsystem "/3(Power_opt)

== system wind_turbine_modified/Wind Turbine Doubly-Fed Induction Generator (Phasor Type)1/Generator & Converters/Control/wind_dfig_rotor/Priority Idr ==
  Idqr* : Inport
  Cartesian to Polar : simulink_extras/Transformations/Cartesian to Polar
  Demux : Demux  Outputs=2
      settings: DisplayOption=none
  Irotor_max^2 : Constant
  Math Function : Math  Operator=square  SignedPower=on
  Math Function1 : Math  Operator=sqrt  SignedPower=on
  Mux : Mux  Inputs=2
  Mux1 : Mux  Inputs=2
  Product : Product  InputSameDT=on  SaturateOnIntegerOverflow=on  OutDataTypeStr=Inherit: Same as first input
  Rate Limiter : RateLimiter  RisingSlewLimit=current_slew_rate  FallingSlewLimit=-current_slew_rate
  Sign : Signum  ZeroCross=off
  Sum : Sum  Inputs=|+-  InputSameDT=on  SaturateOnIntegerOverflow=on  OutDataTypeStr=Inherit: Same as first input
  Switch : Switch  Threshold=1
  Terminator : Terminator
  Idqr_ref : Outport  VectorParamsAs1DForOutWhenUnconnected=off
  wires:
  Product/1 -> Mux1/2
  Demux/2 -> Cartesian to Polar/2, Mux/2, Sign/1
  Demux/1 -> Mux1/1, Math Function/1, Cartesian to Polar/1, Mux/1
  Cartesian to Polar/2 -> Terminator/1
  Cartesian to Polar/1 -> Switch/2
  Mux/1 -> Switch/3
  Irotor_max^2/1 -> Sum/1
  Math Function/1 -> Sum/2
  Sum/1 -> Math Function1/1
  Mux1/1 -> Switch/1
  Switch/1 -> Rate Limiter/1
  Math Function1/1 -> Product/2
  Sign/1 -> Product/1
  Rate Limiter/1 -> Idqr_ref/1
  Idqr*/1 -> Demux/1

== system wind_turbine_modified/Wind Turbine Doubly-Fed Induction Generator (Phasor Type)1/Generator & Converters/Control/wind_dfig_rotor/Q Regulator ==
  Q_ref : Inport
  Q_B1 : Inport  Port=2
  Idr_init : Inport  Port=3
  Enable : EnablePort  PropagateVarSize=During execution  ZeroCross=off
  Mean Value : Subsystem  mask(Mean value){Period=1/Fnom}
      mask prompts: Period "Averaging period (s):"
      mask help: This block uses the running window averaging technique to compute the mean value of the input signal over the specified period.
  Rate Limiter : RateLimiter  RisingSlewLimit=current_slew_rate  FallingSlewLimit=-current_slew_rate
  "Rate Limiter " : RateLimiter  RisingSlewLimit=Q_slew_rate  FallingSlewLimit=-Q_slew_rate
  Subsystem1 : Subsystem  mask{Kp=Kp_Q, Ki=Ki_Q, Limits=[1 -1]}
      mask prompts: Kp "Proportional gain (Kp):"; Ki "Integral gain (Ki):"; Limits "Output limits [Upper Lower]:"
      mask init:
      | Upper_Limit=Limits(1);
      | Lower_Limit=Limits(2);
      mask Display: disp('PI')
  Sum : Sum  Inputs=|+-  InputSameDT=on  SaturateOnIntegerOverflow=on  OutDataTypeStr=Inherit: Same as first input
  Idr* : Outport  VectorParamsAs1DForOutWhenUnconnected=off
  wires:
  Subsystem1/1(Out1) -> Rate Limiter/1  "Idr*"
  Sum/1 -> Subsystem1/1(In1)
  Q_ref/1 -> "Rate Limiter "/1
  Rate Limiter/1 -> Idr*/1
  "Rate Limiter "/1 -> Mean Value/2(Init), Sum/1
  Q_B1/1 -> Mean Value/1(In)
  Mean Value/1(Mean) -> Sum/2
  Idr_init/1 -> Subsystem1/2(Init)

== system wind_turbine_modified/Wind Turbine Doubly-Fed Induction Generator (Phasor Type)1/Generator & Converters/Control/wind_dfig_rotor/V Regulator ==
  V_ref : Inport
  V_B1 : Inport  Port=2
  Idr_init : Inport  Port=3
  Idq_stator : Inport  Port=4
  Idq_grid_conv : Inport  Port=5
  Enable : EnablePort  PropagateVarSize=During execution  ZeroCross=off
  Droop : Gain  Gain=Xs  SaturateOnIntegerOverflow=on  OutDataTypeStr=Inherit: Same as input  ParamDataTypeStr=Inherit: Same as input
  Mean Value : Subsystem  mask(Mean value){Period=1/Fnom}
      mask prompts: Period "Averaging period (s):"
      mask help: This block uses the running window averaging technique to compute the mean value of the input signal over the specified period.
  Mean Value1 : Subsystem  mask(Mean value){Period=1/Fnom}
      mask prompts: Period "Averaging period (s):"
      mask help: This block uses the running window averaging technique to compute the mean value of the input signal over the specified period.
  Rate Limiter : RateLimiter  RisingSlewLimit=current_slew_rate  FallingSlewLimit=-current_slew_rate
  "Rate Limiter " : RateLimiter  RisingSlewLimit=V_slew_rate  FallingSlewLimit=-V_slew_rate
  Selector1 : Selector  InputPortWidth=2  IndexOptions=Index vector (dialog)  Indices=2  OutputSizes=1
  Selector2 : Selector  InputPortWidth=2  IndexOptions=Index vector (dialog)  Indices=2  OutputSizes=1
  Subsystem1 : Subsystem  mask{Kp=Kp_volt_reg, Ki=Ki_volt_reg, Limits=[1 -1]}
      mask prompts: Kp "Proportional gain (Kp):"; Ki "Integral gain (Ki):"; Limits "Output limits [Upper Lower]:"
      mask init:
      | Upper_Limit=Limits(1);
      | Lower_Limit=Limits(2);
      mask Display: disp('PI')
  Sum : Sum  Inputs=|-+-  InputSameDT=on  SaturateOnIntegerOverflow=on  OutDataTypeStr=Inherit: Same as first input
  Sum1 : Sum  InputSameDT=on  SaturateOnIntegerOverflow=on  OutDataTypeStr=Inherit: Same as first input
  Idr* : Outport  VectorParamsAs1DForOutWhenUnconnected=off
  wires:
  "Rate Limiter "/1 -> Mean Value/2(Init), Sum/2
  Rate Limiter/1 -> Idr*/1
  V_ref/1 -> "Rate Limiter "/1
  Sum/1 -> Subsystem1/1(In1)
  Subsystem1/1(Out1) -> Rate Limiter/1  "Idr*"
  Mean Value/1(Mean) -> Sum/3
  V_B1/1 -> Mean Value/1(In)
  Idq_stator/1 -> Selector1/1
  Idq_grid_conv/1 -> Selector2/1
  Selector1/1 -> Sum1/1
  Selector2/1 -> Sum1/2
  Sum1/1 -> Droop/1
  Droop/1 -> Mean Value1/1(In), Mean Value1/2(Init)
  Idr_init/1 -> Subsystem1/2(Init)
  Mean Value1/1(Mean) -> Sum/1

== system wind_turbine_modified/Wind Turbine Doubly-Fed Induction Generator (Phasor Type)1/Generator & Converters/Control/wind_dfig_rotor/dq --> abc ==
  note: Where Vnom = RMS ph-ph nominal voltage
  note: m = Vnom * 2*sqrt(2/3) / Vdc
  note: Required value for modulation index "m" to obtain 1 pu generated voltage by the converter:
  Vdq* : Inport
  Vdc : Inport  Port=2
  Angle : Inport  Port=3
  0-1 : Saturate  UpperLimit=1  LowerLimit=0
  Avoid division by zero : Saturate  UpperLimit=1e6  LowerLimit=1e-6
  Cartesian to Polar : simulink_extras/Transformations/Cartesian to Polar
  Demux1 : Demux  Outputs=2
      settings: DisplayOption=none
  K : Constant  Value=Vnom*2*sqrt(2/3)
  Magnitude-Angle to Complex : MagnitudeAngleToComplex
  Product2 : Product  Inputs=**/  InputSameDT=on  SaturateOnIntegerOverflow=on  OutDataTypeStr=Inherit: Same as first input
  Sum : Sum  Inputs=|++  SaturateOnIntegerOverflow=on
  Vdq_ctrl_rotor_conv : Outport  VectorParamsAs1DForOutWhenUnconnected=off
  wires:
  Vdq*/1 -> Demux1/1
  Cartesian to Polar/2 -> Sum/1
  Cartesian to Polar/1 -> Product2/1
  Demux1/2 -> Cartesian to Polar/2
  Demux1/1 -> Cartesian to Polar/1
  Avoid division by zero/1 -> Product2/3
  K/1 -> Product2/2
  Vdc/1 -> Avoid division by zero/1
  Product2/1 -> 0-1/1  "m"
  0-1/1 -> Magnitude-Angle to Complex/1
  Sum/1 -> Magnitude-Angle to Complex/2
  Angle/1 -> Sum/2
  Magnitude-Angle to Complex/1 -> Vdq_ctrl_rotor_conv/1

== system wind_turbine_modified/Wind Turbine Doubly-Fed Induction Generator (Phasor Type)1/Generator & Converters/Control/wind_dfig_grid/Current regulator/Subsystem3 ==
  In1 : Inport
  Gain : Gain  Gain=Ki  SaturateOnIntegerOverflow=on  OutDataTypeStr=Inherit: Same as input  ParamDataTypeStr=Inherit: Same as input
  Gain1 : Gain  Gain=Kp  SaturateOnIntegerOverflow=on  OutDataTypeStr=Inherit: Same as input  ParamDataTypeStr=Inherit: Same as input
  Integrator : Integrator  InitialCondition=Init  LimitOutput=on  UpperSaturationLimit=Upper_Limit  LowerSaturationLimit=Lower_Limit
  Saturation : Saturate  UpperLimit=Upper_Limit  LowerLimit=Lower_Limit
  Sum7 : Sum  InputSameDT=on  SaturateOnIntegerOverflow=on  OutDataTypeStr=Inherit: Same as first input
  Out1 : Outport  VectorParamsAs1DForOutWhenUnconnected=off
  wires:
  Gain/1 -> Integrator/1
  Gain1/1 -> Sum7/1
  Integrator/1 -> Sum7/2
  In1/1 -> Gain1/1, Gain/1
  Sum7/1 -> Saturation/1
  Saturation/1 -> Out1/1

== system wind_turbine_modified/Wind Turbine Doubly-Fed Induction Generator (Phasor Type)1/Generator & Converters/Control/wind_dfig_grid/DC bus voltage Regulator/Subsystem1 ==
  In1 : Inport
  Gain : Gain  Gain=Ki  SaturateOnIntegerOverflow=on  OutDataTypeStr=Inherit: Same as input  ParamDataTypeStr=Inherit: Same as input
  Gain1 : Gain  Gain=Kp  SaturateOnIntegerOverflow=on  OutDataTypeStr=Inherit: Same as input  ParamDataTypeStr=Inherit: Same as input
  Integrator : Integrator  InitialCondition=Init  LimitOutput=on  UpperSaturationLimit=Upper_Limit  LowerSaturationLimit=Lower_Limit
  Saturation : Saturate  UpperLimit=Upper_Limit  LowerLimit=Lower_Limit
  Sum7 : Sum  InputSameDT=on  SaturateOnIntegerOverflow=on  OutDataTypeStr=Inherit: Same as first input
  Out1 : Outport  VectorParamsAs1DForOutWhenUnconnected=off
  wires:
  Gain/1 -> Integrator/1
  Gain1/1 -> Sum7/1
  Integrator/1 -> Sum7/2
  In1/1 -> Gain1/1, Gain/1
  Sum7/1 -> Saturation/1
  Saturation/1 -> Out1/1

== system wind_turbine_modified/Wind Turbine Doubly-Fed Induction Generator (Phasor Type)1/Generator & Converters/Control/wind_dfig_rotor/Current Regulator/Subsystem1 ==
  In1 : Inport
  Gain : Gain  Gain=Ki  SaturateOnIntegerOverflow=on  OutDataTypeStr=Inherit: Same as input  ParamDataTypeStr=Inherit: Same as input
  Gain1 : Gain  Gain=Kp  SaturateOnIntegerOverflow=on  OutDataTypeStr=Inherit: Same as input  ParamDataTypeStr=Inherit: Same as input
  Integrator : Integrator  InitialCondition=Init  LimitOutput=on  UpperSaturationLimit=Upper_Limit  LowerSaturationLimit=Lower_Limit
  Saturation : Saturate  UpperLimit=Upper_Limit  LowerLimit=Lower_Limit
  Sum7 : Sum  InputSameDT=on  SaturateOnIntegerOverflow=on  OutDataTypeStr=Inherit: Same as first input
  Out1 : Outport  VectorParamsAs1DForOutWhenUnconnected=off
  wires:
  Gain/1 -> Integrator/1
  Gain1/1 -> Sum7/1
  Integrator/1 -> Sum7/2
  In1/1 -> Gain1/1, Gain/1
  Sum7/1 -> Saturation/1
  Saturation/1 -> Out1/1

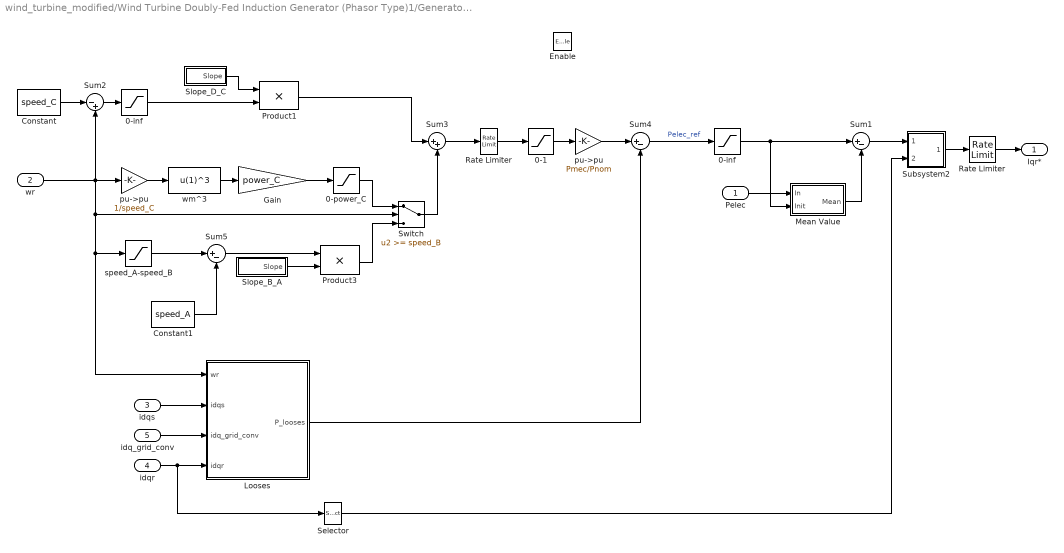
== system wind_turbine_modified/Wind Turbine Doubly-Fed Induction Generator (Phasor Type)1/Generator & Converters/Control/wind_dfig_rotor/Power Regulator/Subsystem ==
  Pelec : Inport
  wr : Inport  Port=2
  idqs : Inport  Port=3
  idqr : Inport  Port=4
  idq_grid_conv : Inport  Port=5
  Enable : EnablePort  PropagateVarSize=During execution
  0-1 : Saturate  UpperLimit=1  LowerLimit=0
  0-inf : Saturate  UpperLimit=inf  LowerLimit=0
  "0-inf " : Saturate  UpperLimit=inf  LowerLimit=0
  0-power_C : Saturate  UpperLimit=power_C  LowerLimit=0
  Constant : Constant  Value=speed_C
  Constant1 : Constant  Value=speed_A
  "Gain " : Gain  Gain=power_C  SaturateOnIntegerOverflow=on  OutDataTypeStr=Inherit: Same as input  ParamDataTypeStr=Inherit: Same as input
  Looses : Subsystem
  Mean Value : Subsystem  mask(Mean value){Period=1/Fnom}
      mask prompts: Period "Averaging period (s):"
      mask help: This block uses the running window averaging technique to compute the mean value of the input signal over the specified period.
  Product1 : Product  SaturateOnIntegerOverflow=on  OutDataTypeStr=Inherit: Same as first input
  Product3 : Product  SaturateOnIntegerOverflow=on  OutDataTypeStr=Inherit: Same as first input
  Rate Limiter : RateLimiter  RisingSlewLimit=current_slew_rate  FallingSlewLimit=-current_slew_rate
  "Rate Limiter " : RateLimiter  RisingSlewLimit=power_slew_rate  FallingSlewLimit=-power_slew_rate
  Selector : Selector  InputPortWidth=2  IndexOptions=Index vector (dialog)  Indices=2  OutputSizes=1
  Slope_B_A : Subsystem
  Slope_D_C : Subsystem
  Subsystem2 : Subsystem  mask{Kp=Kp_power_reg, Ki=Ki_power_reg, Limits=[1 0]}
      mask prompts: Kp "Proportional gain (Kp):"; Ki "Integral gain (Ki):"; Limits "Output limits [Upper Lower]:"
      mask init:
      | Upper_Limit=Limits(1);
      | Lower_Limit=Limits(2);
      mask Display: disp('PI')
  Sum1 : Sum  Inputs=|+-  SaturateOnIntegerOverflow=on
  Sum2 : Sum  Inputs=|-+  SaturateOnIntegerOverflow=on
  Sum3 : Sum  Inputs=|++  SaturateOnIntegerOverflow=on
  Sum4 : Sum  Inputs=|+-  SaturateOnIntegerOverflow=on
  Sum5 : Sum  Inputs=|+-  SaturateOnIntegerOverflow=on
  Switch : Switch  Threshold=speed_B  InputSameDT=off
  "pu->pu " : Gain  Gain=1/speed_C  SaturateOnIntegerOverflow=on  OutDataTypeStr=Inherit: Same as input  ParamDataTypeStr=Inherit: Same as input
  "pu->pu  " : Gain  Gain=Pmec/Pnom  SaturateOnIntegerOverflow=on  OutDataTypeStr=Inherit: Same as input  ParamDataTypeStr=Inherit: Same as input
  speed_A-speed_B : Saturate  UpperLimit=speed_B  LowerLimit=speed_A
  wm^3 : Fcn  Expr=u(1)^3
  Iqr* : Outport  VectorParamsAs1DForOutWhenUnconnected=off
  wires:
  "0-inf "/1 -> Sum1/1, Mean Value/2(Init)
  Slope_B_A/1(Slope) -> Product3/2
  Slope_D_C/1(Slope) -> Product1/1
  Switch/1 -> Sum3/2
  Sum5/1 -> Product3/1
  speed_A-speed_B/1 -> Sum5/1
  Constant1/1 -> Sum5/2
  Product3/1 -> Switch/3
  0-power_C/1 -> Switch/1
  wr/1 -> Switch/2, Looses/1(wr), speed_A-speed_B/1, Sum2/2, "pu->pu "/1
  0-1/1 -> "pu->pu  "/1
  "Rate Limiter "/1 -> 0-1/1
  "pu->pu  "/1 -> Sum4/1
  Sum3/1 -> "Rate Limiter "/1
  Rate Limiter/1 -> Iqr*/1
  "pu->pu "/1 -> wm^3/1
  wm^3/1 -> "Gain "/1
  Sum4/1 -> "0-inf "/1  "Pelec_ref"
  idqs/1 -> Looses/2(idqs)
  idqr/1 -> Looses/4(idqr), Selector/1
  idq_grid_conv/1 -> Looses/3(idq_grid_conv)
  Pelec/1 -> Mean Value/1(In)
  Looses/1(P_looses) -> Sum4/2
  Sum1/1 -> Subsystem2/1(In1)
  Subsystem2/1(Out1) -> Rate Limiter/1
  Selector/1 -> Subsystem2/2(Init)
  Mean Value/1(Mean) -> Sum1/2
  "Gain "/1 -> 0-power_C/1
  Constant/1 -> Sum2/1
  Sum2/1 -> 0-inf/1
  0-inf/1 -> Product1/2
  Product1/1 -> Sum3/1

== system wind_turbine_modified/Wind Turbine Doubly-Fed Induction Generator (Phasor Type)1/Generator & Converters/Control/wind_dfig_rotor/Power Regulator/Subsystem  ==
  Pelec : Inport
  idqr : Inport  Port=2
  Power_opt : Inport  Port=3
  Enable : EnablePort  PropagateVarSize=During execution
  Mean Value : Subsystem  mask(Mean value){Period=1/Fnom}
      mask prompts: Period "Averaging period (s):"
      mask help: This block uses the running window averaging technique to compute the mean value of the input signal over the specified period.
  Rate Limiter : RateLimiter  RisingSlewLimit=current_slew_rate  FallingSlewLimit=-current_slew_rate
  Selector : Selector  InputPortWidth=2  IndexOptions=Index vector (dialog)  Indices=2  OutputSizes=1
  Subsystem2 : Subsystem  mask{Kp=Kp_power_reg, Ki=Ki_power_reg, Limits=[1 0]}
      mask prompts: Kp "Proportional gain (Kp):"; Ki "Integral gain (Ki):"; Limits "Output limits [Upper Lower]:"
      mask init:
      | Upper_Limit=Limits(1);
      | Lower_Limit=Limits(2);
      mask Display: disp('PI')
  Sum1 : Sum  Inputs=|+-  SaturateOnIntegerOverflow=on
  Iqr* : Outport  VectorParamsAs1DForOutWhenUnconnected=off
  wires:
  Rate Limiter/1 -> Iqr*/1
  Sum1/1 -> Subsystem2/1(In1)
  Pelec/1 -> Mean Value/1(In)
  Selector/1 -> Subsystem2/2(Init)
  Power_opt/1 -> Sum1/1, Mean Value/2(Init)
  Subsystem2/1(Out1) -> Rate Limiter/1
  idqr/1 -> Selector/1
  Mean Value/1(Mean) -> Sum1/2
